simulink model "SimplePendulum"  (Simulink 7.7)
settings: Solver=ode45  StartTime=0.0  StopTime=T  RelTol=1e-3
values from neighbouring files (symbols this model uses):
  b = 1    [pendulum.m]    (also in pendulum1.m = 0.5; pendulum2.m = 0; pendulum3.m = 0; pendulum4.m = 0)
  g = 9.8    [pendulum.m]    (also in pendulum1.m; pendulum2.m; pendulum3.m; pendulum4.m)
  J = mp*l^2/12    (= 0.00375)    [pendulum.m]    (also in pendulum1.m; pendulum2.m; pendulum3.m; pendulum4.m)
  mp = 0.5    [pendulum.m]    (also in pendulum1.m; pendulum2.m; pendulum3.m; pendulum4.m)
  r = l/2    (= 0.15)    [pendulum1.m]    (also in pendulum2.m; pendulum3.m; pendulum4.m; pendulum5.m)
  theta0 = pi - pi/8    (= 2.74889357189)    [pendulum.m]    (also in pendulum1.m = 3.09159265359; pendulum2.m = 1.57079632679; pendulum3.m = 1.57079632679; pendulum4.m = 1.57079632679)
  uBar = 0    [pendulum1.m]
settings Model: Creator=mauricio  LastModifiedBy=mauricio
settings DebuggingCC: SolverPrmCheckMsg=none

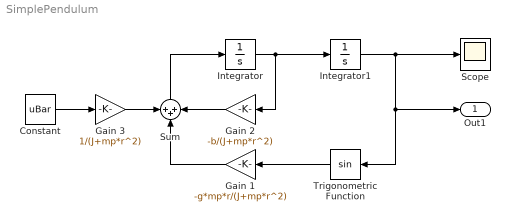
== system SimplePendulum ==
  Constant : Constant  Value=uBar
  Gain 1 : Gain  Gain=-g*mp*r/(J+mp*r^2)
  Gain 2 : Gain  Gain=-b/(J+mp*r^2)
  Gain 3 : Gain  Gain=1/(J+mp*r^2)
  Integrator : Integrator
  Integrator1 : Integrator  InitialCondition=theta0
  Scope : Scope
      settings: YMin=-3.141592653589793  YMax=3.141592653589793
  Sum : Sum  Inputs=+++
  Trigonometric Function : Trigonometry
  Out1 : Outport
  wires:
  Integrator/1 -> Integrator1/1, Gain 2/1
  Integrator1/1 -> Scope/1, Trigonometric Function/1, Out1/1
  Trigonometric Function/1 -> Gain 1/1
  Sum/1 -> Integrator/1
  Gain 3/1 -> Sum/1
  Gain 1/1 -> Sum/2
  Gain 2/1 -> Sum/3
  Constant/1 -> Gain 3/1
